simulink model "q_rotflex"  (R2020a)
settings: Solver=ode1  StartTime=0.0  StopTime=inf  FixedStep=0.002  RelTol=1e-3  EnableMultiTasking=on
values from neighbouring files (symbols this model uses):
  K = [0 0 0 0]    [d_pole_placement_student.m]
undefined symbols (not defined in the file or in its folder): HIL, K_AMP, K_ENC, K_POT, qc_get_step_size, VMAX_AMP, wcf_1, wcf_2
libraries: quarc_library x7, simulink_extras x3
settings Model: SimulationMode=external  ExtModeTrigDuration=10000  Creator=MLevis  LastModifiedBy=MLevis
settings SolverCC: PositivePriorityOrder=on
settings DataIOCC: LimitDataPoints=on  SaveFormat=Array  SignalLoggingSaveFormat=ModelDataLogs  ReturnWorkspaceOutputs=off
settings OptimizationCC: ExpressionDepthLimit=2147483647  InitFltsAndDblsToZero=on
settings DebuggingCC: SaveWithParameterizedLinksMsg=none  UnderspecifiedInitializationDetection=Classic  MergeDetectMultiDrivingBlocksExec=none  SolverPrmCheckMsg=warning  FcnCallInpInsideContextMsg=warning  StateNameClashWarn=warning  SFUnexpectedBacktrackingDiag=warning  SFNoUnconditionalDefaultTransitionDiag=warning  SFExecutionAtInitializationDiag=none  ArithmeticOperatorsInVariantConditions=warning
settings ModelReferenceCC: PropagateSignalLabelsOutOfModel=off
settings RTWCC: Description=QUARC Win64 Target  SystemTargetFile=quarc_win64.tlc  TemplateMakefile=quarc_default_tmf  BuildConfiguration=Faster Runs
settings CodeAppCC: StateflowObjectComments=on
settings STFCustomTargetCC: TargetPreCompLibLocation=C:\PROGRA~3\QUARC\lib\2020a\win64\release  ConcurrentExecutionCompliant=on  GRTInterface=on  SystemTargetFile=quarc_win64.tlc
settings GRTTargetCC: TargetPreCompLibLocation=C:\PROGRA~3\QUARC\lib\2020a\win64\release  TargetLangStandard=C89/C90 (ANSI)  ParMdlRefBuildCompliant=off  CompOptLevelCompliant=off  CombineOutputUpdateFcns=off  MatFileLogging=off  CPPClassGenCompliant=off  GRTInterface=on  UseToolchainInfoCompliant=off  ExtMode=on  ExtModeMexFile=quarc_comm
settings ConfigComp: CovMetricSettings=dw  CovHtmlReporting=on  CovSaveCumulativeToWorkspaceVar=on  CovSaveSingleToWorkspaceVar=on

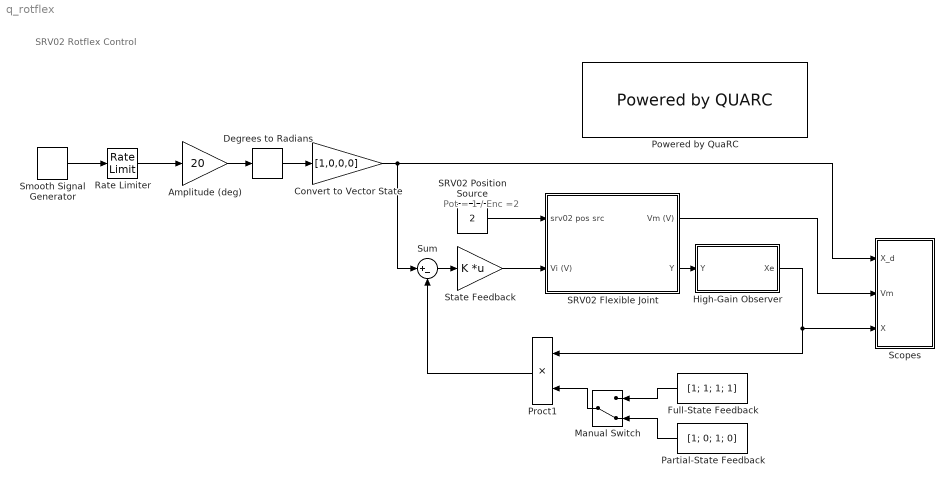
== system q_rotflex ==
  note: SRV02 Rotflex Control
  note: Pot = 1 / Enc =2
  Amplitude (deg) : Gain  Gain=20  SaturateOnIntegerOverflow=on  OutDataTypeStr=Inherit: Same as input  ParamDataTypeStr=Inherit: Same as input
  Convert to Vector State : Gain  Gain=[1,0,0,0]
  Degrees to Radians : simulink_extras/Transformations/Degrees to Radians
  Full-State Feedback : Constant  Value=[1; 1; 1; 1]
  High-Gain Observer : Subsystem
  Manual Switch : ManualSwitch  CurrentSetting=0
  Partial-State Feedback : Constant  Value=[1; 0; 1; 0]
  Powered by QuaRC : quarc_library/Logos/Powered by QUARC
  Proct1 : Product  InputSameDT=on  RndMeth=Zero  SaturateOnIntegerOverflow=on  OutDataTypeStr=Inherit: Same as first input
  Rate Limiter : RateLimiter  RisingSlewLimit=100  FallingSlewLimit=-100  SampleTimeMode=inherited
  SRV02 Flexible Joint : Subsystem
  SRV02 Position Source : Constant  Value=2
  Scopes : Subsystem
  Smooth Signal Generator : quarc_library/Sources/Signals/Smooth Signal Generator  signal_type=Square  source=Internal (dialog parameters)  amplitude=1  frequency=0.33  initial_phase=-pi  sample_time=qc_get_step_size  output_cos=off
      settings: SourceProductName=QUARC Targets
  State Feedback : Gain  Gain=K  Multiplication=Matrix(K*u)  SaturateOnIntegerOverflow=on  OutDataTypeStr=Inherit: Same as input  ParamDataTypeStr=Inherit: Same as input
  Sum : Sum  Inputs=|+-
  wires:
  High-Gain Observer/1(Xe) -> Scopes/3(X), Proct1/1
  SRV02 Flexible Joint/2(Y) -> High-Gain Observer/1(Y)
  SRV02 Flexible Joint/1(Vm (V)) -> Scopes/2(Vm)
  Sum/1 -> State Feedback/1
  State Feedback/1 -> SRV02 Flexible Joint/2(Vi (V))
  Degrees to Radians/1 -> Convert to Vector State/1
  Convert to Vector State/1 -> Sum/1, Scopes/1(X_d)
  Amplitude (deg)/1 -> Degrees to Radians/1
  Rate Limiter/1 -> Amplitude (deg)/1
  Manual Switch/1 -> Proct1/2
  Proct1/1 -> Sum/2
  SRV02 Position Source/1 -> SRV02 Flexible Joint/1(srv02 pos src)
  Smooth Signal Generator/1 -> Rate Limiter/1
  Full-State Feedback/1 -> Manual Switch/1
  Partial-State Feedback/1 -> Manual Switch/2

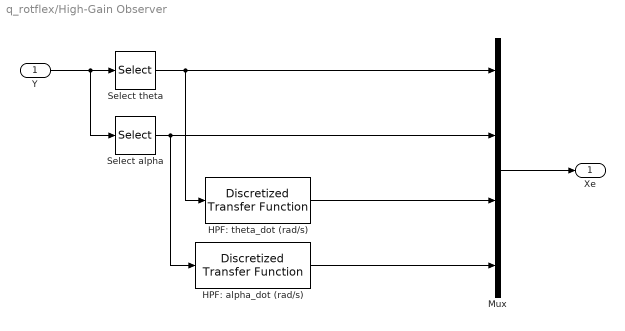
== system q_rotflex/High-Gain Observer ==
  Y : Inport
  HPF: alpha_dot (rad/s) : quarc_library/Discrete/Discretized Transfer Function  num=[wcf_2 0]  den=[1 wcf_2]  method=tustin  Ts=qc_get_step_size
      settings: SourceProductName=QUARC Targets
  HPF: theta_dot (rad/s) : quarc_library/Discrete/Discretized Transfer Function  num=[wcf_1 0]  den=[1 wcf_1]  method=tustin  Ts=qc_get_step_size
      settings: SourceProductName=QUARC Targets
  Mux : Mux
  Select alpha : Selector  InputPortWidth=2  IndexOptions=Index vector (dialog)  Indices=2  OutputSizes=1
  Select theta : Selector  InputPortWidth=2  IndexOptions=Index vector (dialog)  Indices=1  OutputSizes=1
  Xe : Outport
  wires:
  Select alpha/1 -> Mux/2, HPF: alpha_dot (rad/s)/1
  Mux/1 -> Xe/1
  Y/1 -> Select alpha/1, Select theta/1
  HPF: theta_dot (rad/s)/1 -> Mux/3
  Select theta/1 -> Mux/1, HPF: theta_dot (rad/s)/1
  HPF: alpha_dot (rad/s)/1 -> Mux/4

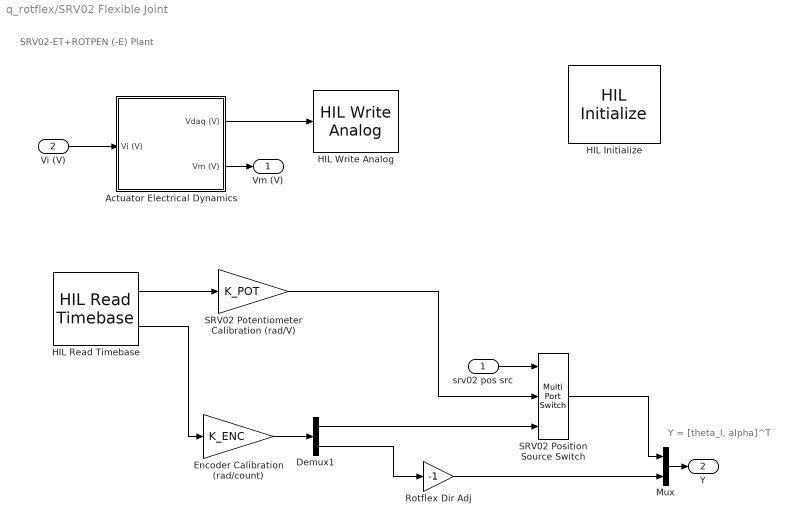
== system q_rotflex/SRV02 Flexible Joint ==
  note: SRV02-ET+ROTPEN (-E) Plant
  note: Y = [theta_l, alpha]^T
  srv02 pos src : Inport
  Vi (V) : Inport  Port=2
  Actuator Electrical Dynamics : Subsystem
  Demux1 : Demux  Outputs=2
  Encoder Calibration (rad/count) : Gain  Gain=K_ENC  SaturateOnIntegerOverflow=on  OutDataTypeStr=Inherit: Same as input  ParamDataTypeStr=Inherit: Same as input
  HIL Initialize : quarc_library/Data Acquisition/Generic/Configuration/HIL Initialize  object_name=HIL-1  board_type=q2_usb  board_number=0  board_options=d0=digital;d1=digital;led=auto;update_rate=normal;decimation=1  exclusive=off  active=on  hardware_clocks=[0]  clock_modes=[]  initial_clock_frequencies=[]  set_clock_params_at_start=off  set_clock_params_at_switch_in=off  set_clock_frequencies_at_start=off  set_clock_frequencies_at_switch_in=off  analog_input_channels=[0:1]  analog_input_configurations=[]  analog_input_maximums=10  analog_input_minimums=-10  set_analog_input_params_at_start=on  set_analog_input_params_at_switch_in=off  analog_output_channels=[0:1]  analog_output_maximums=10  analog_output_minimums=-10  initial_analog_outputs=[0]  final_analog_outputs=[0]  watchdog_analog_outputs=0  set_analog_output_params_at_start=on  set_analog_output_params_at_switch_in=off  set_analog_outputs_at_start=on  set_analog_outputs_at_switch_in=off  set_analog_outputs_at_terminate=on  set_analog_outputs_at_switch_out=off  set_analog_outputs_on_watchdog=off  digital_input_channels=[]  digital_output_channels=[]  digital_output_configuration=[]  initial_digital_outputs=[1]  final_digital_outputs=[1]  watchdog_digital_outputs=[1]  set_digital_output_params_at_start=off  set_digital_output_params_at_switch_in=off  set_digital_outputs_at_start=on  set_digital_outputs_at_switch_in=off  set_digital_outputs_at_terminate=on  set_digital_outputs_at_switch_out=off  set_digital_outputs_on_watchdog=off  encoder_channels=[0:1]  quadrature=[4]  encoder_filter_frequency=[]  initial_encoder_counts=[0]  set_encoder_params_at_start=on  set_encoder_params_at_switch_in=off  set_encoder_counts_at_start=on  set_encoder_counts_at_switch_in=off  pwm_channels=[]  pwm_modes=[0]  pwm_frequency=1/0.020  pwm_configuration=[]  pwm_alignment=[]  pwm_polarity=[]  pwm_leading_deadband=[]  pwm_trailing_deadband=[]  initial_pwm_outputs=[0]  final_pwm_outputs=[0]  watchdog_pwm_outputs=[0]  set_pwm_params_at_start=on  set_pwm_params_at_switch_in=off  set_pwm_outputs_at_start=on  set_pwm_outputs_at_switch_in=off  set_pwm_outputs_at_terminate=on  set_pwm_outputs_at_switch_out=off  set_pwm_outputs_on_watchdog=off  other_output_channels=[]  initial_other_outputs=[]  final_other_outputs=[]  watchdog_other_outputs=[]  set_other_outputs_at_start=off  set_other_outputs_at_switch_in=off  set_other_outputs_at_terminate=off  set_other_outputs_at_switch_out=off  set_other_outputs_on_watchdog=off
  HIL Read Timebase : quarc_library/Data Acquisition/Generic/Timebases/HIL Read Timebase  object_name=HIL-1  clock=0  analog_channels=[0]  encoder_channels=[0:1]  digital_channels=[]  other_channels=[]  active=on  vector_output=on  data_type_mode=Inherit via back propagation  encoder_data_type=double  digital_data_type=boolean  overflow_mode=Error on overflow  samples_in_buffer=max(ceil(1/qc_get_step_size), 1)
  HIL Write Analog : quarc_library/Data Acquisition/Generic/Immediate I//O/HIL Write Analog  object_name=HIL-1  channels=0  sample_time=-1  active=off  vector_input=off
  Mux : Mux  Inputs=2
  Rotflex Dir Adj : Gain  Gain=-1
  SRV02 Position Source Switch : MultiPortSwitch  Inputs=2
  SRV02 Potentiometer Calibration (rad/V) : Gain  Gain=K_POT  SaturateOnIntegerOverflow=on  OutDataTypeStr=Inherit: Same as input  ParamDataTypeStr=Inherit: Same as input
  Vm (V) : Outport  InitialOutput=0
  Y : Outport  Port=2  InitialOutput=0
  wires:
  SRV02 Potentiometer Calibration (rad/V)/1 -> SRV02 Position Source Switch/2
  HIL Read Timebase/1 -> SRV02 Potentiometer Calibration (rad/V)/1
  Demux1/1 -> SRV02 Position Source Switch/3
  Encoder Calibration (rad/count)/1 -> Demux1/1
  HIL Read Timebase/2 -> Encoder Calibration (rad/count)/1
  srv02 pos src/1 -> SRV02 Position Source Switch/1
  Actuator Electrical Dynamics/1(Vdaq (V)) -> HIL Write Analog/1
  SRV02 Position Source Switch/1 -> Mux/1
  Rotflex Dir Adj/1 -> Mux/2
  Mux/1 -> Y/1
  Demux1/2 -> Rotflex Dir Adj/1
  Actuator Electrical Dynamics/2(Vm (V)) -> Vm (V)/1
  Vi (V)/1 -> Actuator Electrical Dynamics/1(Vi (V))

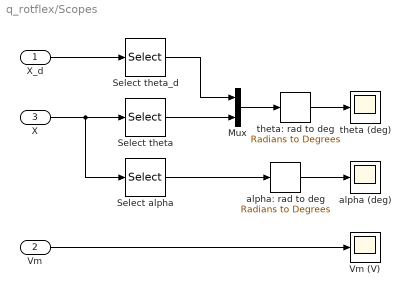
== system q_rotflex/Scopes ==
  X_d : Inport
  Vm : Inport  Port=2
  X : Inport  Port=3
  Mux : Mux  Inputs=2
  Select alpha : Selector  InputPortWidth=4  IndexOptions=Index vector (dialog)  Indices=2  OutputSizes=1
  Select theta : Selector  InputPortWidth=4  IndexOptions=Index vector (dialog)  Indices=1  OutputSizes=1
  Select theta_d : Selector  InputPortWidth=4  IndexOptions=Index vector (dialog)  Indices=1  OutputSizes=1
  Vm (V) : Scope
  alpha (deg) : Scope
  alpha: rad to deg : simulink_extras/Transformations/Radians to Degrees
  theta (deg) : Scope
  theta: rad to deg : simulink_extras/Transformations/Radians to Degrees
  wires:
  Vm/1 -> Vm (V)/1
  X_d/1 -> Select theta_d/1
  Mux/1 -> theta: rad to deg/1
  Select alpha/1 -> alpha: rad to deg/1
  Select theta/1 -> Mux/2
  alpha: rad to deg/1 -> alpha (deg)/1
  X/1 -> Select alpha/1, Select theta/1
  Select theta_d/1 -> Mux/1
  theta: rad to deg/1 -> theta (deg)/1

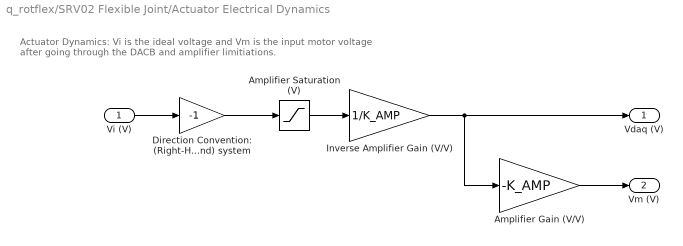
== system q_rotflex/SRV02 Flexible Joint/Actuator Electrical Dynamics ==
  note: Actuator Dynamics: Vi is the ideal voltage and Vm is the
      | input motor voltage after going through the DACB and amplifier limitiations.
  Vi (V) : Inport
  Amplifier Gain (V/V) : Gain  Gain=-K_AMP
  Amplifier Saturation (V) : Saturate  UpperLimit=VMAX_AMP  LowerLimit=-VMAX_AMP
  Direction Convention: (Right-Hand) system : Gain  Gain=-1  SaturateOnIntegerOverflow=on  OutDataTypeStr=Inherit: Same as input  ParamDataTypeStr=Inherit: Same as input
  Inverse Amplifier Gain (V/V) : Gain  Gain=1/K_AMP
  Vdaq (V) : Outport
  Vm (V) : Outport  Port=2
  wires:
  Direction Convention: (Right-Hand) system/1 -> Amplifier Saturation (V)/1
  Amplifier Gain (V/V)/1 -> Vm (V)/1
  Inverse Amplifier Gain (V/V)/1 -> Vdaq (V)/1, Amplifier Gain (V/V)/1
  Amplifier Saturation (V)/1 -> Inverse Amplifier Gain (V/V)/1
  Vi (V)/1 -> Direction Convention: (Right-Hand) system/1
